simulink model "parallel_force_pos_control"  (R2021b)
settings: Solver=FixedStepAuto  StartTime=0.0  StopTime=10  FixedStep=Ts  RelTol=1e-3
undefined symbols (not defined in the file): dqi, fd, invMd, K, KD, KF, KI, KP, Md, myRobot, qf, qi, qr, xd, xr
settings Model: Creator=simon  LastModifiedBy=luigi
settings SolverCC: ZeroCrossControl=DisableAll  AlgebraicLoopSolver=TrustRegion
settings DebuggingCC: SFMachineParentedDataDiag=warning

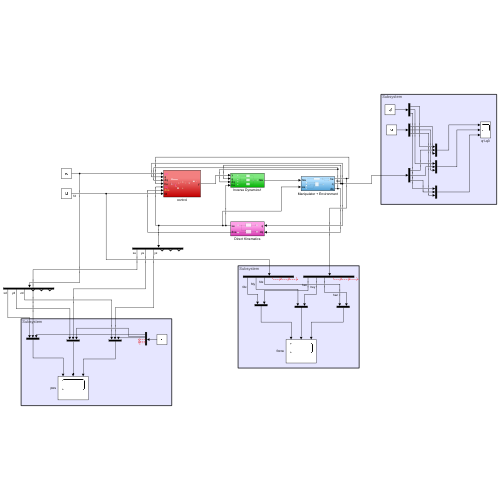
[thumbnail: Simulink's stored preview of the top-level diagram]
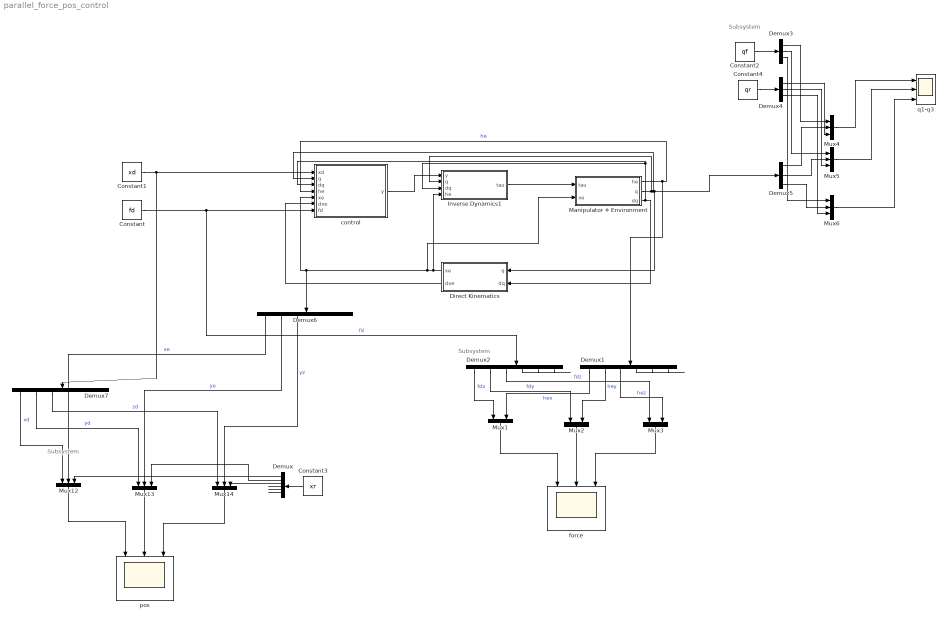
== system parallel_force_pos_control ==
  note: Subsystem
  note: Subsystem
  note: Subsystem
  Constant : Constant  Value=fd
  Constant1 : Constant  Value=xd
  Constant2 : Constant  Value=qf
  Constant3 : Constant  Value=xr
  Constant4 : Constant  Value=qr
  Demux{,1..2,6..7} (5 alike) : Demux  Outputs=6
  Demux3 : Demux  Outputs=3
  Demux4 : Demux  Outputs=3
  Demux5 : Demux  Outputs=myRobot.N
  Direct Kinematics : Subsystem
  Inverse Dynamics1 : Subsystem
  Manipulator + Environment : Subsystem
  Mux1 : Mux  Inputs=2
  Mux{4..6,12..14} (6 alike) : Mux  Inputs=3
  Mux2 : Mux  Inputs=2
  Mux3 : Mux  Inputs=2
  control : Subsystem
  force : Scope  NumInputPorts=3
  pos : Scope  NumInputPorts=3
  q1-q3 : Scope  NumInputPorts=3
  wires:
  Manipulator + Environment/3(dq) -> control/3(dq), Inverse Dynamics1/3(dq), Direct Kinematics/2(dq)
  Manipulator + Environment/1(he) -> Demux1/1, control/4(he)  "he"
  Direct Kinematics/1(xe) -> control/5(xe), Demux6/1, Manipulator + Environment/2(xe), Inverse Dynamics1/4(he)
  Constant/1 -> Demux2/1, control/7(fd)  "fd"
  Constant1/1 -> Demux7/1, control/1(xd)
  Direct Kinematics/2(dxe) -> control/6(dxe)
  control/1(y) -> Inverse Dynamics1/1(y)
  Inverse Dynamics1/1(tau) -> Manipulator + Environment/1(tau)
  Demux7/1 -> Mux12/1  "xd"
  Demux7/2 -> Mux13/1  "yd"
  Demux7/3 -> Mux14/1  "zd"
  Demux6/1 -> Mux12/2  "xe"
  Demux6/2 -> Mux13/2  "ye"
  Demux6/3 -> Mux14/2  "yz"
  Demux/6 -> ?
  Demux/2 -> Mux13/3
  Demux/3 -> Mux14/3
  Demux/1 -> Mux12/3
  Constant3/1 -> Demux/1
  Mux13/1 -> pos/2
  Demux/5 -> ?
  Mux12/1 -> pos/1
  Demux/4 -> ?
  Mux14/1 -> pos/3
  Demux1/6 -> ?
  Demux2/6 -> ?
  Demux2/5 -> ?
  Demux1/4 -> ?
  Demux1/5 -> ?
  Demux2/4 -> ?
  Demux1/3 -> Mux3/2  "hez"
  Mux1/1 -> force/1
  Demux1/2 -> Mux2/2  "hey"
  Demux2/2 -> Mux2/1  "fdy"
  Mux3/1 -> force/3
  Demux2/3 -> Mux3/1  "fdz"
  Mux2/1 -> force/2
  Demux1/1 -> Mux1/2  "hex"
  Demux2/1 -> Mux1/1  "fdx"
  Manipulator + Environment/2(q) -> Demux5/1, Direct Kinematics/1(q), control/2(q), Inverse Dynamics1/2(q)
  Mux5/1 -> q1-q3/2
  Demux3/1 -> Mux4/1
  Demux4/1 -> Mux4/3
  Constant4/1 -> Demux4/1
  Demux5/2 -> Mux5/2
  Demux4/2 -> Mux5/3
  Mux4/1 -> q1-q3/1
  Demux5/1 -> Mux4/2
  Demux4/3 -> Mux6/3
  Mux6/1 -> q1-q3/3
  Constant2/1 -> Demux3/1
  Demux5/3 -> Mux6/2
  Demux3/3 -> Mux6/1
  Demux3/2 -> Mux5/1

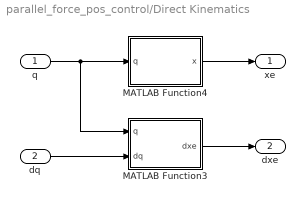
== system parallel_force_pos_control/Direct Kinematics ==
  q : Inport
  dq : Inport  Port=2
  MATLAB Function3 : MATLAB Function  TreatAsAtomicUnit=on
  MATLAB Function4 : MATLAB Function  TreatAsAtomicUnit=on
  xe : Outport
  dxe : Outport  Port=2
  wires:
  q/1 -> MATLAB Function3/1(q), MATLAB Function4/1(q)
  MATLAB Function4/1(x) -> xe/1
  dq/1 -> MATLAB Function3/2(dq)
  MATLAB Function3/1(dxe) -> dxe/1

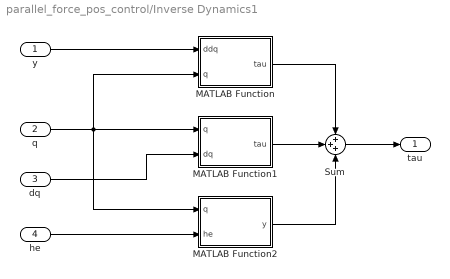
== system parallel_force_pos_control/Inverse Dynamics1 ==
  y : Inport
  q : Inport  Port=2
  dq : Inport  Port=3
  he : Inport  Port=4
  MATLAB Function : MATLAB Function  TreatAsAtomicUnit=on
  MATLAB Function1 : MATLAB Function  TreatAsAtomicUnit=on
  MATLAB Function2 : MATLAB Function  TreatAsAtomicUnit=on
  Sum : Sum  Inputs=+++
  tau : Outport
  wires:
  MATLAB Function2/1(y) -> Sum/3
  y/1 -> MATLAB Function/1(ddq)
  dq/1 -> MATLAB Function1/2(dq)
  he/1 -> MATLAB Function2/2(he)
  Sum/1 -> tau/1
  MATLAB Function/1(tau) -> Sum/1
  q/1 -> MATLAB Function1/1(q), MATLAB Function2/1(q), MATLAB Function/2(q)
  MATLAB Function1/1(tau) -> Sum/2

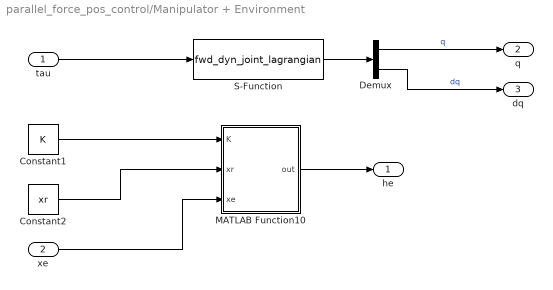
== system parallel_force_pos_control/Manipulator + Environment ==
  tau : Inport
  xe : Inport  Port=2
  Constant1 : Constant  Value=K
  Constant2 : Constant  Value=xr
  Demux : Demux  Outputs=2
  MATLAB Function10 : MATLAB Function  TreatAsAtomicUnit=on
  S-Function : S-Function  FunctionName=fwd_dyn_joint_lagrangian  Parameters=myRobot,qi,dqi  SFunctionDeploymentMode=off  EnableBusSupport=off
  he : Outport
  q : Outport  Port=2
  dq : Outport  Port=3
  wires:
  Constant2/1 -> MATLAB Function10/2(xr)
  Constant1/1 -> MATLAB Function10/1(K)
  Demux/1 -> q/1  "q"
  MATLAB Function10/1(out) -> he/1
  S-Function/1 -> Demux/1
  tau/1 -> S-Function/1
  xe/1 -> MATLAB Function10/3(xe)
  Demux/2 -> dq/1  "dq"

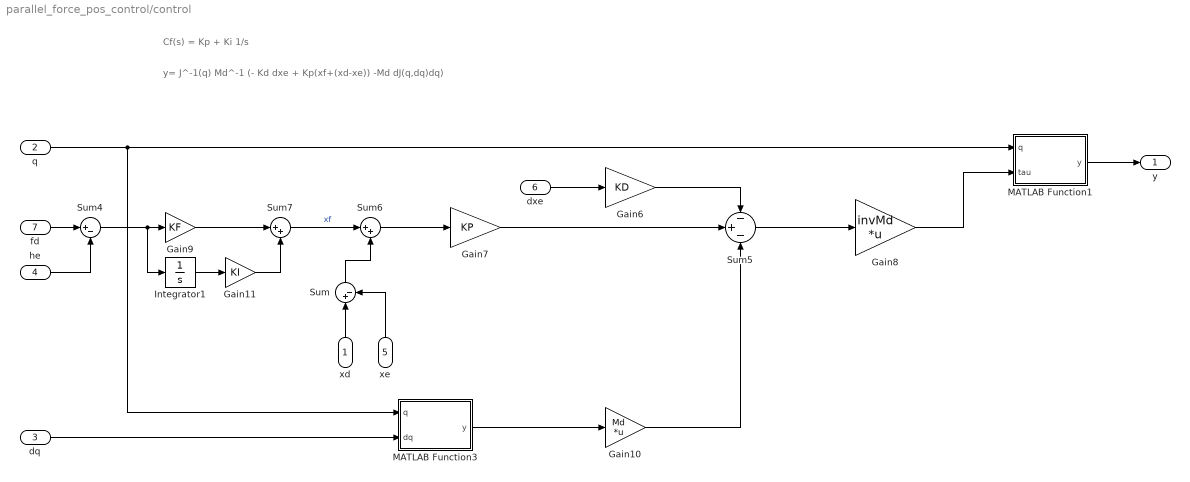
== system parallel_force_pos_control/control ==
  note: y= J^-1(q) Md^-1 (- Kd dxe + Kp(xf+(xd-xe)) -Md dJ(q,dq)dq)
  note: Cf(s) = Kp + Ki 1/s
  xd : Inport
  q : Inport  Port=2
  dq : Inport  Port=3
  he : Inport  Port=4
  xe : Inport  Port=5
  dxe : Inport  Port=6
  fd : Inport  Port=7
  Gain10 : Gain  Gain=Md  Multiplication=Matrix(K*u)
  Gain11 : Gain  Gain=KI
  Gain6 : Gain  Gain=KD
  Gain7 : Gain  Gain=KP
  Gain8 : Gain  Gain=invMd  Multiplication=Matrix(K*u)
  Gain9 : Gain  Gain=KF
  Integrator1 : Integrator
  MATLAB Function1 : MATLAB Function  TreatAsAtomicUnit=on
  MATLAB Function3 : MATLAB Function  TreatAsAtomicUnit=on
  Sum : Sum  Inputs=|+-
  Sum4 : Sum  Inputs=|+-
  Sum5 : Sum  Inputs=-+-
  Sum6 : Sum  Inputs=|++
  Sum7 : Sum  Inputs=|++
  y : Outport
  wires:
  Gain7/1 -> Sum5/2
  q/1 -> MATLAB Function3/1(q), MATLAB Function1/1(q)
  Sum7/1 -> Sum6/1  "xf"
  Gain11/1 -> Sum7/2
  Gain9/1 -> Sum7/1
  Sum5/1 -> Gain8/1
  Sum4/1 -> Integrator1/1, Gain9/1
  Gain6/1 -> Sum5/1
  dq/1 -> MATLAB Function3/2(dq)
  fd/1 -> Sum4/1
  Gain10/1 -> Sum5/3
  Integrator1/1 -> Gain11/1
  dxe/1 -> Gain6/1
  Sum6/1 -> Gain7/1
  he/1 -> Sum4/2
  MATLAB Function1/1(y) -> y/1
  Gain8/1 -> MATLAB Function1/2(tau)
  MATLAB Function3/1(y) -> Gain10/1
  xe/1 -> Sum/2
  xd/1 -> Sum/1
  Sum/1 -> Sum6/2

== matlab function parallel_force_pos_control/Inverse Dynamics1/MATLAB Function2 ==
  data: q input; he input; y output
function y = fcn(q, he)
y = getJ(q)'*he;

== matlab function parallel_force_pos_control/control/MATLAB Function1 ==
  data: q input; y output; tau input
function y = invJ(q, tau)

y = getInvJ(q)*tau;

== matlab function parallel_force_pos_control/control/MATLAB Function3 ==
  data: q input; y output; dq input
function y = dJa(q, dq)

y = getDiffJa(q,dq)*dq;

== matlab function parallel_force_pos_control/Direct Kinematics/MATLAB Function3 ==
  data: q input; dxe output; dq input
function dxe = Ja(q, dq)

dxe = getJa(q)*dq;

== matlab function parallel_force_pos_control/Direct Kinematics/MATLAB Function4 ==
  data: q input; x output
function x = k(q)

x = getK(q);

== matlab function parallel_force_pos_control/Inverse Dynamics1/MATLAB Function ==
  data: ddq input size=3; q input size=3; tau output
function tau = B(ddq, q)

tau = getB(q)*ddq;

== matlab function parallel_force_pos_control/Inverse Dynamics1/MATLAB Function1 ==
  data: q input size=3; tau output; dq input size=3
function tau = n(q, dq)

tau = getN(q, dq);

== matlab function parallel_force_pos_control/Manipulator + Environment/MATLAB Function10 ==
  data: K input; out output size=6; xr input; xe input size=6
function out = hde(K,xr, xe)
%consider the interaction only in z direction
if xe(3) < xr(3) 
    out = K*(xe-xr);
else 
    out = zeros(6,1);
end
